simulink model "MotorXploer"  (R2025a)
settings: Solver=FixedStepAuto  StartTime=0.0  StopTime=inf  FixedStep=0.001  RelTol=1e-3  EnableMultiTasking=on
values from neighbouring files (symbols this model uses):
  Chirmp_Time = 20.5    [Cross_Validation.m]
  Mode = 5    [Cross_Validation.m]
  Ramp_Slope = 0.05    [Cross_Validation.m]
  Sine_Freq = pi/4    (= 0.785398163397)    [Cross_Validation.m]
  Stair_Wait = 0.5    [Cross_Validation.m]
  Step_Value = 1    [Cross_Validation.m]
undefined symbols (not defined in the file or in its folder): Blocking, LF, Non
libraries: amg_usbconverter_n_connect_lib x3, simulink x2
settings Model: Creator=beamk  LastModifiedBy=ACER
settings OptimizationCC: DefaultParameterBehavior=Inlined  EnhancedBackFolding=on  PassReuseOutputArgsAs=Individual arguments  ZeroExternalMemoryAtStartup=off  ZeroInternalMemoryAtStartup=off  MaxStackSize=64  OptimizeBlockOrder=speed  DifferentSizesBufferReuse=on  OptimizationCustomize=off  EfficientTunableParamExpr=on
settings DebuggingCC: ParameterTunabilityLossMsg=error
settings HardwareCC: ProdBitPerPointer=32.0  ProdBitPerSizeT=32.0  ProdBitPerPtrDiffT=32.0  ProdLargestAtomicInteger=Long  ProdLargestAtomicFloat=Double  ProdWordSize=32.0  ProdLongLongMode=on  ProdHWDeviceType=ARM Compatible->ARM Cortex-M
settings SFSimCC: MATLABDynamicMemAlloc=off
settings RTWCC: SystemTargetFile=ert.tlc  HardwareBoard=STM32G4xx Based  TemplateMakefile=ert_default_tmf  Toolchain=Armclang Compiler  Description=Embedded Coder
settings CodeAppCC: ForceParamTrailComments=on  IgnoreCustomStorageClasses=off  OperatorAnnotations=on  SimulinkDataObjDesc=on  SFDataObjDesc=on  InsertBlockDesc=on
settings ERTTargetCC: ExtModeTransport=3.0  ExtModeStaticAllocSize=2048.0  TargetLangStandard=C99 (ISO)  CodeReplacementLibrary=ARM Cortex-M

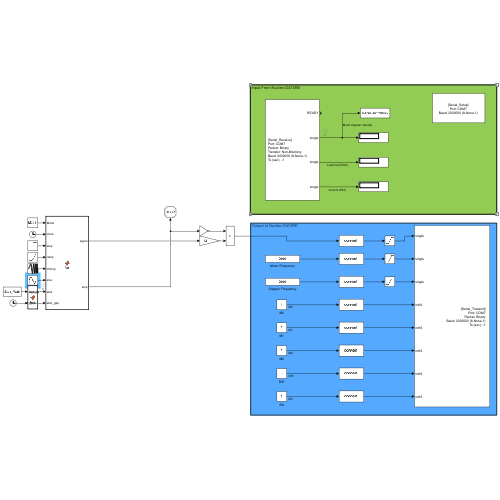
[thumbnail: Simulink's stored preview of the top-level diagram]
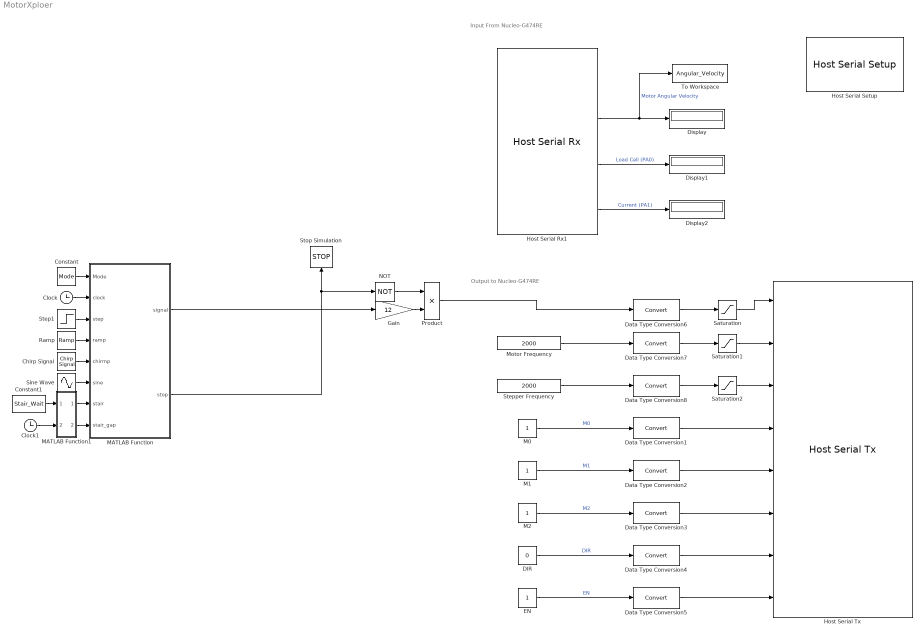
== system MotorXploer ==
  note: Output to Nucleo-G474RE
  note: Input From Nucleo-G474RE
  Chirp Signal : simulink/Sources/Chirp Signal  f1=0  T=Chirmp_Time  f2=Chirmp_Freq
  Clock : Clock
  Clock1 : Clock
  Constant : Constant  Value=Mode
  Constant1 : Constant  Value=Stair_Wait
  DIR : Constant  Value=0
  Data Type Conversion{1..8} (8 alike) : DataTypeConversion  SaturateOnIntegerOverflow=off  RndMeth=Floor
  Display : Display
  Display1 : Display
  Display2 : Display
  EN : Constant
  Gain : Gain  Gain=12
  Host Serial Rx1 : amg_usbconverter_n_connect_lib/Host Serial Rx  conf=rx  port=<auto>  baudrate=2000000  databits=8  parity=None  stopbit=1  flowcontrol=None  transfer=Non-Blocking  timeout=5  packetmode=Binary  enableinitialvalues=off  initialvalues=[]  binheader='25'  binterminator='4E'  porttype_double=0  porttype_single=3  porttype_int8=0  porttype_uint8=0  porttype_int16=0  porttype_uint16=0  porttype_int32=0  porttype_uint32=0  asciiformat='%f,%f,%d,%d'  rx_asciiterminator="LF (0x0A - \"\\n\")"  tx_asciiterminator="CRLF (0x0D 0x0A - \"\\r\\n\")"  sampletime=-1  enablecustomportlabel=off  cinputportlabel=0  coutputportlabel=A  portpinstr=0  blockid=HostSerialRx1  inputporttype=[]  inputportwidth=[]  inputportlabel={}  outputporttype=[3 1 1 1]  outputportwidth=[1 1 1 1]  outputportlabel={'READY','single','single','single'}  compat=0  optionstring=[]  autoport='COM7'
  Host Serial Setup : amg_usbconverter_n_connect_lib/Host Serial Setup  conf=setup  port=<auto>  baudrate=2000000  databits=8  parity=None  stopbit=1  flowcontrol=None  transfer=Blocking  timeout=2  packetmode=Binary  initialvalues=[]  binheader='7E 7E'  binterminator='03 03'  porttype_double=0  porttype_single=1  porttype_int8=0  porttype_uint8=0  porttype_int16=0  porttype_uint16=0  porttype_int32=0  porttype_uint32=2  asciiformat='%d %u %x'  rx_asciiterminator="CRLF (0x0D 0x0A - \"\\r\\n\")"  tx_asciiterminator="CRLF (0x0D 0x0A - \"\\r\\n\")"  sampletime=-1  enablecustomportlabel=off  cinputportlabel=0  coutputportlabel=A  portpinstr=0  blockid=HostSerialSetup  inputporttype=[]  inputportwidth=[]  inputportlabel={}  outputporttype=[]  outputportwidth=[]  outputportlabel={}  compat=0  optionstring=[]  autoport='COM7'
  Host Serial Tx : amg_usbconverter_n_connect_lib/Host Serial Tx  conf=tx  port=<auto>  baudrate=2000000  databits=8  parity=None  stopbit=1  flowcontrol=None  transfer=Blocking  timeout=2  packetmode=Binary  initialvalues=[]  binheader='25'  binterminator='4E'  porttype_double=0  porttype_single=3  porttype_int8=0  porttype_uint8=0  porttype_int16=5  porttype_uint16=0  porttype_int32=0  porttype_uint32=0  asciiformat='%d,%f'  rx_asciiterminator="CRLF (0x0D 0x0A - \"\\r\\n\")"  tx_asciiterminator="CRLF (0x0D 0x0A - \"\\r\\n\")"  sampletime=-1  enablecustomportlabel=off  cinputportlabel=0  coutputportlabel=A  portpinstr=0  blockid=HostSerialTx  inputporttype=[1 1 1 4 4 4 4 4]  inputportwidth=[1 1 1 1 1 1 1 1]  inputportlabel={'single','single','single','int16','int16','int16','int16','int16'}  outputporttype=[]  outputportwidth=[]  outputportlabel={}  compat=0  optionstring=[]  autoport='COM7'
      settings: SourceProductName=aMG USB Converter N
  M0 : Constant
  M1 : Constant
  M2 : Constant
  MATLAB Function : MATLAB Function  TreatAsAtomicUnit=on
  MATLAB Function1 : MATLAB Function  TreatAsAtomicUnit=on
  Motor Frequency : Constant  Value=2000  OutDataTypeStr=single
  NOT : Logic  Operator=NOT  IconShape=distinctive  AllPortsSameDT=off  OutDataTypeStr=boolean
  Product : Product
  Ramp : simulink/Sources/Ramp  slope=Ramp_Slope  start=0.5  InitialOutput=0
  Saturation : Saturate  UpperLimit=65535  LowerLimit=-65535
  Saturation1 : Saturate  UpperLimit=20000  LowerLimit=0
  Saturation2 : Saturate  UpperLimit=inf  LowerLimit=0
  Sine Wave : Sin  Frequency=Sine_Freq  SampleTime=0
  Step1 : Step  Time=0.5  After=Step_Value  SampleTime=0
  Stepper Frequency : Constant  Value=2000  OutDataTypeStr=single
  Stop Simulation : Stop
  To Workspace : ToWorkspace  VariableName=Angular_Velocity  SaveFormat=Structure With Time  SampleTime=-1
  wires:
  Host Serial Rx1/2 -> To Workspace/1, Display/1  "Motor Angular Velocity"
  Host Serial Rx1/3 -> Display1/1  "Load Cell (PA0)"
  M0/1 -> Data Type Conversion1/1  "M0"
  EN/1 -> Data Type Conversion5/1  "EN"
  DIR/1 -> Data Type Conversion4/1  "DIR"
  M1/1 -> Data Type Conversion2/1  "M1"
  M2/1 -> Data Type Conversion3/1  "M2"
  Motor Frequency/1 -> Data Type Conversion7/1
  Stepper Frequency/1 -> Data Type Conversion8/1
  Data Type Conversion1/1 -> Host Serial Tx/4
  Data Type Conversion2/1 -> Host Serial Tx/5
  Data Type Conversion3/1 -> Host Serial Tx/6
  Data Type Conversion4/1 -> Host Serial Tx/7
  Data Type Conversion5/1 -> Host Serial Tx/8
  Data Type Conversion6/1 -> Saturation/1
  Saturation/1 -> Host Serial Tx/1
  Data Type Conversion7/1 -> Saturation1/1
  Data Type Conversion8/1 -> Saturation2/1
  Saturation1/1 -> Host Serial Tx/2
  Saturation2/1 -> Host Serial Tx/3
  Host Serial Rx1/4 -> Display2/1  "Current (PA1)"
  Ramp/1 -> MATLAB Function/4(ramp)
  Constant/1 -> MATLAB Function/1(Mode)
  NOT/1 -> Product/1
  Step1/1 -> MATLAB Function/3(step)
  Chirp Signal/1 -> MATLAB Function/5(chirmp)
  MATLAB Function/2(stop) -> NOT/1, Stop Simulation/1
  MATLAB Function1/1(signal) -> MATLAB Function/7(stair)
  Clock/1 -> MATLAB Function/2(clock)
  Clock1/1 -> MATLAB Function1/2(clock)
  Constant1/1 -> MATLAB Function1/1(stair_gap)
  Sine Wave/1 -> MATLAB Function/6(sine)
  Gain/1 -> Product/2
  MATLAB Function/1(signal) -> Gain/1
  MATLAB Function1/2(stair_gaps) -> MATLAB Function/8(stair_gap)
  Product/1 -> Data Type Conversion6/1

== matlab function MotorXploer/MATLAB Function1 ==
  data: signal output; stair_gaps output; stair_gap input; clock input
function [signal,stair_gaps]= fcn(stair_gap,clock)
time_offset = 0.5;
All_signal = 0.1:0.1:1;
clock_usage = clock - time_offset;
if clock_usage < 0
    clock_usage = 0;
end
phase = fix(clock_usage/stair_gap/2);
stair_gaps = stair_gap;
if clock < 0.5
    signal = 0;
    return;
end

if phase <= 9
    buffer = clock_usage - 2*stair_gap*phase;
    if buffer < stair_gap
        signal = All_signal(phase+1);
    else
        signal = 0;
    end
else
    signal = 0;
end

    end

== matlab function MotorXploer/MATLAB Function ==
  data: Mode input; signal output; clock input; step input; ramp input; chirmp input; sine input; stair input; stop output; stair_gap input
function [signal, stop] = fcn(Mode, clock, step, ramp, chirmp, sine, stair, stair_gap)

% Default outputs
signal = 0;
stop   = 0;

% Initial 0.5 sec zero output
if clock < 0.5
    return;
end

switch Mode

    case 1   % STEP
        signal = step;
        if clock >= 10.5
            stop = 1;
        end

    case 2   % RAMP
        signal = ramp;
        if signal >= 1
            stop = 1;
        end

    case 3   % CHIRP
        signal = chirmp;
        if clock >= 10.5
            stop = 1;
        end

    case 4   % SINE
        signal = sine;
        if clock >= 10.5
            stop = 1;
        end

  case 5   % STAIR
        signal = stair;

        % 10 amplitudes × (ON + OFF) × stair_gap + 0.5 sec initial
        total_time = 0.6 + 20 * stair_gap;

        if clock >= total_time
            stop = 1;
        end

    otherwise
        signal = 0;
        stop   = 0;
end

end
